simulink model "Model"  (R2020b)
settings: Solver=VariableStepAuto  StartTime=0.0  StopTime=20  MaxStep=0.1  RelTol=1e-1
values from neighbouring files (symbols this model uses):
  D = [0 ... (first row only)    [Data_clean.m]
  g = 9.81    [Data_clean.m]
  k_cart = 0.0113    [Data_clean.m]
  L = 5    [Data_clean.m]
  m = 12000    [Data_clean.m]
  M = 1000    [Data_clean.m]
  Ts = 0.1    [Data_clean.m]
undefined symbols (not defined in the file or in its folder): blk, Discrete, iA, isLTV, lastPcov, lastu, lastx, MDscale, mpc1_plant, MVscale, nCC, nu, nud, nv, nxp, ny, nym, p, RMVscale, Time, ts, uoff, X, xoff, Y, Yscale, Z
libraries: sm_lib x76, mpcsigdimcheck_private x76, nesl_utility x12, ctrlSharedLib x8, simulink_extras x5, mpclib x1
(part 5 of 8)

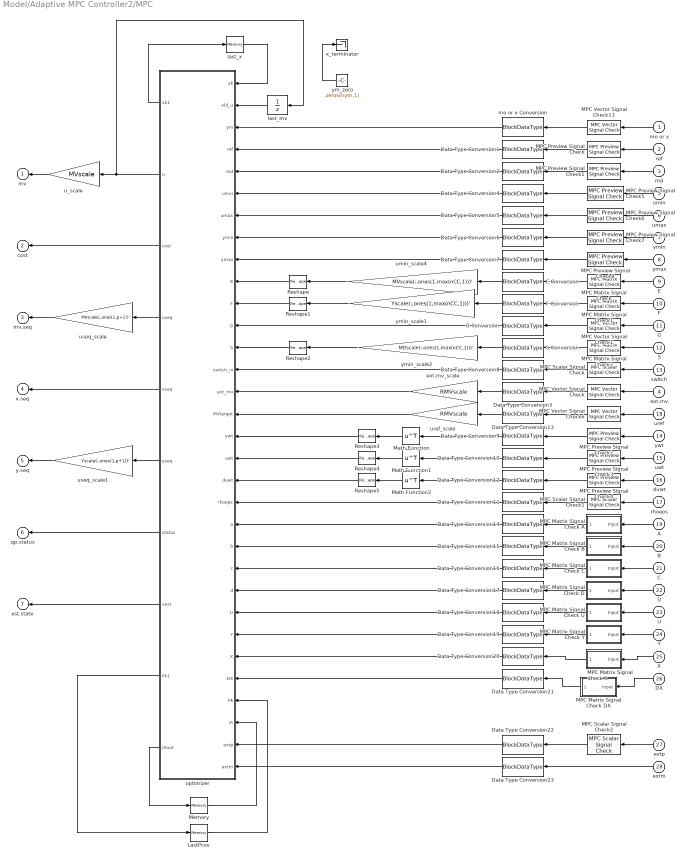
== system Model/Adaptive MPC Controller2/MPC ==
  mo or x : Inport
  ref : Inport  Port=2
  md : Inport  Port=3
  ext.mv : Inport  Port=4
  umin : Inport  Port=5
  umax : Inport  Port=6
  ymin : Inport  Port=7
  ymax : Inport  Port=8
  E : Inport  Port=9
  F : Inport  Port=10
  G : Inport  Port=11
  S : Inport  Port=12
  switch : Inport  Port=13
  ywt : Inport  Port=14
  uwt : Inport  Port=15
  duwt : Inport  Port=16
  rhoeps : Inport  Port=17
  uref : Inport  Port=18
  A : Inport  Port=19
  B : Inport  Port=20
  C : Inport  Port=21
  D : Inport  Port=22
  U : Inport  Port=23
  Y : Inport  Port=24
  X : Inport  Port=25
  DX : Inport  Port=26
  extp : Inport  Port=27
  extm : Inport  Port=28
  Data Type Conversion{1..23} (23 alike) : DataTypeConversion  OutDataTypeStr=BlockDataType
  E Conversion : DataTypeConversion  OutDataTypeStr=BlockDataType
  F Conversion : DataTypeConversion  OutDataTypeStr=BlockDataType
  G Conversion : DataTypeConversion  OutDataTypeStr=BlockDataType
  LastPcov : Memory  InitialCondition=lastPcov  InheritSampleTime=on  LinearizeAsDelay=on
  MPC Matrix Signal Check : mpcsigdimcheck_private/MPC Matrix Signal Check  blockname=blk  signalname='CustomConstraint.E'  numrow=max(nCC,1)  numcol=nu  steps=0  isLTV=0
      settings: SourceProductBaseCode=MP
  MPC Matrix Signal Check A : Subsystem  AncestorBlock=mpcsigdimcheck_private/MPC Matrix Signal Check  mask(MPCSignalDimensionCheck){blockname=blk, signalname='Model.A', numrow=nxp, numcol=nxp, steps=p, isLTV=isLTV}
      mask prompts: blockname "Block name"; signalname "Signal name"; numrow "Number of rows"; numcol "Number of columns"; steps "Number of prediction steps"; isLTV "Linear Time-Varying (LTV) plants"
      mask help: Internal use to check MPC input signal dimensions at compile time.
      mask init:
      | nrow = uint16(numrow);
      | ncol = uint16(numcol);
      | nsteps = uint16(steps);
      | isltv = uint16(isLTV);
  MPC Matrix Signal Check B : Subsystem  AncestorBlock=mpcsigdimcheck_private/MPC Matrix Signal Check  mask(MPCSignalDimensionCheck){blockname=blk, signalname='Model.B', numrow=nxp, numcol=nu+nv-1+nud, steps=p, isLTV=isLTV}
      mask prompts: blockname "Block name"; signalname "Signal name"; numrow "Number of rows"; numcol "Number of columns"; steps "Number of prediction steps"; isLTV "Linear Time-Varying (LTV) plants"
      mask help: Internal use to check MPC input signal dimensions at compile time.
      mask init:
      | nrow = uint16(numrow);
      | ncol = uint16(numcol);
      | nsteps = uint16(steps);
      | isltv = uint16(isLTV);
  MPC Matrix Signal Check C : Subsystem  AncestorBlock=mpcsigdimcheck_private/MPC Matrix Signal Check  mask(MPCSignalDimensionCheck){blockname=blk, signalname='Model.C', numrow=ny, numcol=nxp, steps=p, isLTV=isLTV}
      mask prompts: blockname "Block name"; signalname "Signal name"; numrow "Number of rows"; numcol "Number of columns"; steps "Number of prediction steps"; isLTV "Linear Time-Varying (LTV) plants"
      mask help: Internal use to check MPC input signal dimensions at compile time.
      mask init:
      | nrow = uint16(numrow);
      | ncol = uint16(numcol);
      | nsteps = uint16(steps);
      | isltv = uint16(isLTV);
  MPC Matrix Signal Check D : Subsystem  AncestorBlock=mpcsigdimcheck_private/MPC Matrix Signal Check  mask(MPCSignalDimensionCheck){blockname=blk, signalname='Model.D', numrow=ny, numcol=nu+nv-1+nud, steps=p, isLTV=isLTV}
      mask prompts: blockname "Block name"; signalname "Signal name"; numrow "Number of rows"; numcol "Number of columns"; steps "Number of prediction steps"; isLTV "Linear Time-Varying (LTV) plants"
      mask help: Internal use to check MPC input signal dimensions at compile time.
      mask init:
      | nrow = uint16(numrow);
      | ncol = uint16(numcol);
      | nsteps = uint16(steps);
      | isltv = uint16(isLTV);
  MPC Matrix Signal Check DX : Subsystem  AncestorBlock=mpcsigdimcheck_private/MPC Matrix Signal Check  mask(MPCSignalDimensionCheck){blockname=blk, signalname='Model.DX', numrow=nxp, numcol=1, steps=p, isLTV=isLTV}
      mask prompts: blockname "Block name"; signalname "Signal name"; numrow "Number of rows"; numcol "Number of columns"; steps "Number of prediction steps"; isLTV "Linear Time-Varying (LTV) plants"
      mask help: Internal use to check MPC input signal dimensions at compile time.
      mask init:
      | nrow = uint16(numrow);
      | ncol = uint16(numcol);
      | nsteps = uint16(steps);
      | isltv = uint16(isLTV);
  MPC Matrix Signal Check U : Subsystem  AncestorBlock=mpcsigdimcheck_private/MPC Matrix Signal Check  mask(MPCSignalDimensionCheck){blockname=blk, signalname='Model.U', numrow=nu+nv-1+nud, numcol=1, steps=p, isLTV=isLTV}
      mask prompts: blockname "Block name"; signalname "Signal name"; numrow "Number of rows"; numcol "Number of columns"; steps "Number of prediction steps"; isLTV "Linear Time-Varying (LTV) plants"
      mask help: Internal use to check MPC input signal dimensions at compile time.
      mask init:
      | nrow = uint16(numrow);
      | ncol = uint16(numcol);
      | nsteps = uint16(steps);
      | isltv = uint16(isLTV);
  MPC Matrix Signal Check X : Subsystem  AncestorBlock=mpcsigdimcheck_private/MPC Matrix Signal Check  mask(MPCSignalDimensionCheck){blockname=blk, signalname='Model.X', numrow=nxp, numcol=1, steps=p, isLTV=isLTV}
      mask prompts: blockname "Block name"; signalname "Signal name"; numrow "Number of rows"; numcol "Number of columns"; steps "Number of prediction steps"; isLTV "Linear Time-Varying (LTV) plants"
      mask help: Internal use to check MPC input signal dimensions at compile time.
      mask init:
      | nrow = uint16(numrow);
      | ncol = uint16(numcol);
      | nsteps = uint16(steps);
      | isltv = uint16(isLTV);
  MPC Matrix Signal Check Y : Subsystem  AncestorBlock=mpcsigdimcheck_private/MPC Matrix Signal Check  mask(MPCSignalDimensionCheck){blockname=blk, signalname='Model.Y', numrow=ny, numcol=1, steps=p, isLTV=isLTV}
      mask prompts: blockname "Block name"; signalname "Signal name"; numrow "Number of rows"; numcol "Number of columns"; steps "Number of prediction steps"; isLTV "Linear Time-Varying (LTV) plants"
      mask help: Internal use to check MPC input signal dimensions at compile time.
      mask init:
      | nrow = uint16(numrow);
      | ncol = uint16(numcol);
      | nsteps = uint16(steps);
      | isltv = uint16(isLTV);
  MPC Matrix Signal Check1 : mpcsigdimcheck_private/MPC Matrix Signal Check  blockname=blk  signalname='CustomConstraint.F'  numrow=max(nCC,1)  numcol=ny  steps=0  isLTV=0
      settings: SourceProductBaseCode=MP
  MPC Matrix Signal Check2 : mpcsigdimcheck_private/MPC Matrix Signal Check  blockname=blk  signalname='CustomConstraint.S'  numrow=max(nCC,1)  numcol=max(nv-1,1)  steps=0  isLTV=0
      settings: SourceProductBaseCode=MP
  MPC Preview Signal Check : mpcsigdimcheck_private/MPC Preview Signal Check  blockname=blk  signalname='ref'  numrow=p  numcol=ny
      settings: SourceProductBaseCode=MP
  MPC Preview Signal Check1 : mpcsigdimcheck_private/MPC Preview Signal Check  blockname=blk  signalname='md'  numrow=p+1  numcol=max(nv-1,1)
      settings: SourceProductBaseCode=MP
  MPC Preview Signal Check2 : mpcsigdimcheck_private/MPC Preview Signal Check  blockname=blk  signalname='y.wt'  numrow=p  numcol=ny
      settings: SourceProductBaseCode=MP
  MPC Preview Signal Check3 : mpcsigdimcheck_private/MPC Preview Signal Check  blockname=blk  signalname='u.wt'  numrow=p  numcol=nu
      settings: SourceProductBaseCode=MP
  MPC Preview Signal Check4 : mpcsigdimcheck_private/MPC Preview Signal Check  blockname=blk  signalname='du.wt'  numrow=p  numcol=nu
      settings: SourceProductBaseCode=MP
  MPC Preview Signal Check5 : mpcsigdimcheck_private/MPC Preview Signal Check  blockname=blk  signalname='umin'  numrow=p  numcol=nu
      settings: SourceProductBaseCode=MP
  MPC Preview Signal Check6 : mpcsigdimcheck_private/MPC Preview Signal Check  blockname=blk  signalname='umax'  numrow=p  numcol=nu
      settings: SourceProductBaseCode=MP
  MPC Preview Signal Check7 : mpcsigdimcheck_private/MPC Preview Signal Check  blockname=blk  signalname='ymin'  numrow=p  numcol=ny
      settings: SourceProductBaseCode=MP
  MPC Preview Signal Check8 : mpcsigdimcheck_private/MPC Preview Signal Check  blockname=blk  signalname='ymax'  numrow=p  numcol=ny
      settings: SourceProductBaseCode=MP
  MPC Scalar Signal Check : mpcsigdimcheck_private/MPC Scalar Signal Check  blockname=blk  signalname='switch'
      settings: SourceProductBaseCode=MP
  MPC Scalar Signal Check1 : mpcsigdimcheck_private/MPC Scalar Signal Check  blockname=blk  signalname='ecr.wt'
      settings: SourceProductBaseCode=MP
  MPC Scalar Signal Check2 : mpcsigdimcheck_private/MPC Scalar Signal Check  blockname=blk  signalname='p'
      settings: SourceProductBaseCode=MP
  MPC Vector Signal Check : mpcsigdimcheck_private/MPC Vector Signal Check  blockname=blk  signalname='ext.mv'  num=nu  vectortype=Any
      settings: SourceProductBaseCode=MP
  MPC Vector Signal Check1 : mpcsigdimcheck_private/MPC Vector Signal Check  blockname=blk  signalname='CustomConstraint.G'  num=max(nCC,1)  vectortype=Column
      settings: SourceProductBaseCode=MP
  MPC Vector Signal Check11 : mpcsigdimcheck_private/MPC Vector Signal Check  blockname=blk  signalname=strmoorx  num=nmoorx  vectortype=Any
      settings: SourceProductBaseCode=MP
  MPC Vector Signal Check6 : mpcsigdimcheck_private/MPC Vector Signal Check  blockname=blk  signalname='mv.target'  num=nu  vectortype=Any
      settings: SourceProductBaseCode=MP
  Math Function : Math  Operator=transpose  SignedPower=on  SaturateOnIntegerOverflow=on
  Math Function1 : Math  Operator=transpose  SignedPower=on  SaturateOnIntegerOverflow=on
  Math Function2 : Math  Operator=transpose  SignedPower=on  SaturateOnIntegerOverflow=on
  Memory : Memory  InitialCondition=iA  InheritSampleTime=on  LinearizeAsDelay=on
  Reshape : Reshape  OutputDimensionality=Customize  OutputDimensions=double([max(nCC,1),nu])
  Reshape1 : Reshape  OutputDimensionality=Customize  OutputDimensions=double([max(nCC,1),ny])
  Reshape2 : Reshape  OutputDimensionality=Customize  OutputDimensions=double([max(nCC,1),max(nv-1,1)])
  Reshape3 : Reshape  OutputDimensionality=Column vector (2-D)
  Reshape4 : Reshape  OutputDimensionality=Column vector (2-D)
  Reshape5 : Reshape  OutputDimensionality=Column vector (2-D)
  S Conversion : DataTypeConversion  OutDataTypeStr=BlockDataType
  ext.mv_scale : Gain  Gain=RMVscale  SampleTime=ts
  last_mv : UnitDelay  InitialCondition=lastu+uoff  SampleTime=ts  HasFrameUpgradeWarning=on
  last_x : Memory  InitialCondition=lastx+xoff  InheritSampleTime=on  LinearizeAsDelay=on
  mo or x Conversion : DataTypeConversion  OutDataTypeStr=BlockDataType
  optimizer : Subsystem  Variant=on  VariantControlMode=label  VariantControl=Variant1  LabelModeActiveChoice=FixedHorizon
  u_scale : Gain  Gain=MVscale  SampleTime=ts
  umin_scale4 : Gain  Gain=MVscale(:,ones(1,max(nCC,1)))'  SampleTime=ts
  uref_scale : Gain  Gain=RMVscale  SampleTime=ts
  useq_scale : Gain  Gain=MVscale(:,ones(1,p+1))'  SampleTime=ts
  useq_scale1 : Gain  Gain=Yscale(:,ones(1,p+1))'  SampleTime=ts
  x_terminator : Terminator
  ym_zero : Constant  Value=zeros(nym,1)  OutDataTypeStr=BlockDataType
  ymin_scale1 : Gain  Gain=Yscale(:,ones(1,max(nCC,1)))'  SampleTime=ts
  ymin_scale2 : Gain  Gain=MDscale(:,ones(1,max(nCC,1)))'  SampleTime=ts
  mv : Outport  OutDataTypeStr=BlockDataType  VectorParamsAs1DForOutWhenUnconnected=off
  cost : Outport  Port=2  OutDataTypeStr=BlockDataType  VectorParamsAs1DForOutWhenUnconnected=off
  mv.seq : Outport  Port=3  OutDataTypeStr=BlockDataType  VectorParamsAs1DForOutWhenUnconnected=off
  x.seq : Outport  Port=4  OutDataTypeStr=BlockDataType  VectorParamsAs1DForOutWhenUnconnected=off
  y.seq : Outport  Port=5  OutDataTypeStr=BlockDataType  VectorParamsAs1DForOutWhenUnconnected=off
  qp.status : Outport  Port=6  OutDataTypeStr=BlockDataType  VectorParamsAs1DForOutWhenUnconnected=off
  est.state : Outport  Port=7  OutDataTypeStr=BlockDataType  VectorParamsAs1DForOutWhenUnconnected=off
  wires:
  MPC Scalar Signal Check2/1 -> Data Type Conversion22/1
  extm/1 -> Data Type Conversion23/1
  extp/1 -> MPC Scalar Signal Check2/1
  Data Type Conversion23/1 -> optimizer/32(extm)
  Data Type Conversion22/1 -> optimizer/31(extp)
  optimizer/10(" iAout") -> Memory/1
  optimizer/9(" Pk1") -> LastPcov/1
  optimizer/8(" xest") -> est.state/1
  optimizer/7(" status") -> qp.status/1
  optimizer/6(" yseq") -> useq_scale1/1
  optimizer/5(" xseq") -> x.seq/1
  optimizer/4(" useq") -> useq_scale/1
  optimizer/3(" cost") -> cost/1
  optimizer/2(" u") -> last_mv/1, u_scale/1
  optimizer/1(" xk1") -> last_x/1
  Memory/1 -> optimizer/30("iA ")
  LastPcov/1 -> optimizer/29("Pk ")
  Data Type Conversion21/1 -> optimizer/28("DX ")
  Data Type Conversion20/1 -> optimizer/27("X ")
  Data Type Conversion19/1 -> optimizer/26("Y ")
  Data Type Conversion18/1 -> optimizer/25("U ")
  Data Type Conversion17/1 -> optimizer/24("d ")
  Data Type Conversion16/1 -> optimizer/23("c ")
  Data Type Conversion15/1 -> optimizer/22("b ")
  Data Type Conversion14/1 -> optimizer/21("a ")
  Data Type Conversion11/1 -> optimizer/20("rhoeps ")
  Reshape5/1 -> optimizer/19("duwt ")
  Reshape4/1 -> optimizer/18("uwt ")
  Reshape3/1 -> optimizer/17("ywt ")
  uref_scale/1 -> optimizer/16("MVtarget ")
  ext.mv_scale/1 -> optimizer/15("ext_mv ")
  Data Type Conversion8/1 -> optimizer/14("switch_in ")
  Reshape2/1 -> optimizer/13("S ")
  G Conversion/1 -> optimizer/12("G ")
  Reshape1/1 -> optimizer/11("F ")
  Reshape/1 -> optimizer/10("E ")
  Data Type Conversion7/1 -> optimizer/9("ymax ")
  Data Type Conversion6/1 -> optimizer/8("ymin ")
  Data Type Conversion5/1 -> optimizer/7("umax ")
  Data Type Conversion4/1 -> optimizer/6("umin ")
  Data Type Conversion2/1 -> optimizer/5("md ")
  Data Type Conversion1/1 -> optimizer/4("ref ")
  mo or x Conversion/1 -> optimizer/3("ym ")
  last_mv/1 -> optimizer/2("old_u ")
  last_x/1 -> optimizer/1("xk ")
  useq_scale1/1 -> y.seq/1
  Math Function2/1 -> Reshape5/1
  Math Function1/1 -> Reshape4/1
  Math Function/1 -> Reshape3/1
  MPC Matrix Signal Check1/1 -> F Conversion/1
  umin_scale4/1 -> Reshape/1
  ymin_scale1/1 -> Reshape1/1
  G/1 -> MPC Vector Signal Check1/1
  F/1 -> MPC Matrix Signal Check1/1
  E Conversion/1 -> umin_scale4/1
  ymin_scale2/1 -> Reshape2/1
  MPC Matrix Signal Check/1 -> E Conversion/1
  S/1 -> MPC Matrix Signal Check2/1
  E/1 -> MPC Matrix Signal Check/1
  MPC Matrix Signal Check2/1 -> S Conversion/1
  MPC Vector Signal Check1/1 -> G Conversion/1
  S Conversion/1 -> ymin_scale2/1
  F Conversion/1 -> ymin_scale1/1
  MPC Matrix Signal Check DX/1(Output) -> Data Type Conversion21/1
  MPC Matrix Signal Check X/1(Output) -> Data Type Conversion20/1
  MPC Matrix Signal Check Y/1(Output) -> Data Type Conversion19/1
  MPC Matrix Signal Check U/1(Output) -> Data Type Conversion18/1
  MPC Matrix Signal Check D/1(Output) -> Data Type Conversion17/1
  MPC Matrix Signal Check C/1(Output) -> Data Type Conversion16/1
  MPC Matrix Signal Check B/1(Output) -> Data Type Conversion15/1
  MPC Matrix Signal Check A/1(Output) -> Data Type Conversion14/1
  MPC Scalar Signal Check1/1 -> Data Type Conversion11/1
  MPC Preview Signal Check4/1 -> Data Type Conversion12/1
  MPC Preview Signal Check3/1 -> Data Type Conversion10/1
  MPC Preview Signal Check2/1 -> Data Type Conversion9/1
  MPC Vector Signal Check6/1 -> Data Type Conversion13/1
  MPC Vector Signal Check/1 -> Data Type Conversion3/1
  MPC Scalar Signal Check/1 -> Data Type Conversion8/1
  MPC Preview Signal Check8/1 -> Data Type Conversion7/1
  MPC Preview Signal Check7/1 -> Data Type Conversion6/1
  MPC Preview Signal Check6/1 -> Data Type Conversion5/1
  MPC Preview Signal Check5/1 -> Data Type Conversion4/1
  MPC Preview Signal Check1/1 -> Data Type Conversion2/1
  MPC Preview Signal Check/1 -> Data Type Conversion1/1
  MPC Vector Signal Check11/1 -> mo or x Conversion/1
  useq_scale/1 -> mv.seq/1
  u_scale/1 -> mv/1
  DX/1 -> MPC Matrix Signal Check DX/1(Input)
  X/1 -> MPC Matrix Signal Check X/1(Input)
  Y/1 -> MPC Matrix Signal Check Y/1(Input)
  U/1 -> MPC Matrix Signal Check U/1(Input)
  D/1 -> MPC Matrix Signal Check D/1(Input)
  C/1 -> MPC Matrix Signal Check C/1(Input)
  B/1 -> MPC Matrix Signal Check B/1(Input)
  A/1 -> MPC Matrix Signal Check A/1(Input)
  md/1 -> MPC Preview Signal Check1/1
  umin/1 -> MPC Preview Signal Check5/1
  umax/1 -> MPC Preview Signal Check6/1
  ymin/1 -> MPC Preview Signal Check7/1
  ymax/1 -> MPC Preview Signal Check8/1
  switch/1 -> MPC Scalar Signal Check/1
  ext.mv/1 -> MPC Vector Signal Check/1
  Data Type Conversion3/1 -> ext.mv_scale/1
  ref/1 -> MPC Preview Signal Check/1
  mo or x/1 -> MPC Vector Signal Check11/1
  ywt/1 -> MPC Preview Signal Check2/1
  uwt/1 -> MPC Preview Signal Check3/1
  Data Type Conversion9/1 -> Math Function/1
  Data Type Conversion12/1 -> Math Function2/1
  rhoeps/1 -> MPC Scalar Signal Check1/1
  duwt/1 -> MPC Preview Signal Check4/1
  Data Type Conversion10/1 -> Math Function1/1
  uref/1 -> MPC Vector Signal Check6/1
  Data Type Conversion13/1 -> uref_scale/1
  ym_zero/1 -> x_terminator/1

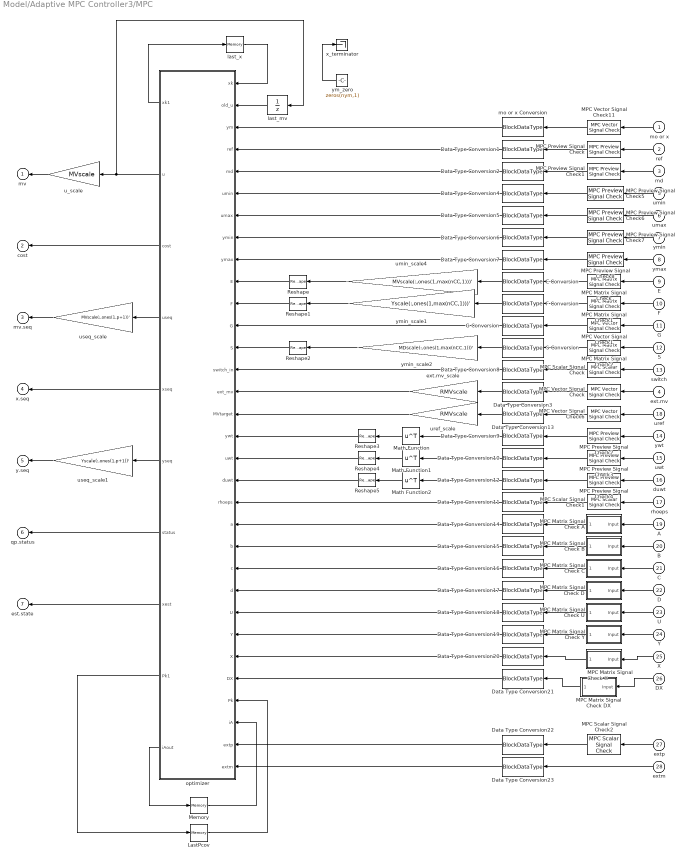
== system Model/Adaptive MPC Controller3/MPC ==
  mo or x : Inport
  ref : Inport  Port=2
  md : Inport  Port=3
  ext.mv : Inport  Port=4
  umin : Inport  Port=5
  umax : Inport  Port=6
  ymin : Inport  Port=7
  ymax : Inport  Port=8
  E : Inport  Port=9
  F : Inport  Port=10
  G : Inport  Port=11
  S : Inport  Port=12
  switch : Inport  Port=13
  ywt : Inport  Port=14
  uwt : Inport  Port=15
  duwt : Inport  Port=16
  rhoeps : Inport  Port=17
  uref : Inport  Port=18
  A : Inport  Port=19
  B : Inport  Port=20
  C : Inport  Port=21
  D : Inport  Port=22
  U : Inport  Port=23
  Y : Inport  Port=24
  X : Inport  Port=25
  DX : Inport  Port=26
  extp : Inport  Port=27
  extm : Inport  Port=28
  Data Type Conversion{1..23} (23 alike) : DataTypeConversion  OutDataTypeStr=BlockDataType
  E Conversion : DataTypeConversion  OutDataTypeStr=BlockDataType
  F Conversion : DataTypeConversion  OutDataTypeStr=BlockDataType
  G Conversion : DataTypeConversion  OutDataTypeStr=BlockDataType
  LastPcov : Memory  InitialCondition=lastPcov  InheritSampleTime=on  LinearizeAsDelay=on
  MPC Matrix Signal Check : mpcsigdimcheck_private/MPC Matrix Signal Check  blockname=blk  signalname='CustomConstraint.E'  numrow=max(nCC,1)  numcol=nu  steps=0  isLTV=0
      settings: SourceProductBaseCode=MP
  MPC Matrix Signal Check A : Subsystem  AncestorBlock=mpcsigdimcheck_private/MPC Matrix Signal Check  mask(MPCSignalDimensionCheck){blockname=blk, signalname='Model.A', numrow=nxp, numcol=nxp, steps=p, isLTV=isLTV}
      mask prompts: blockname "Block name"; signalname "Signal name"; numrow "Number of rows"; numcol "Number of columns"; steps "Number of prediction steps"; isLTV "Linear Time-Varying (LTV) plants"
      mask help: Internal use to check MPC input signal dimensions at compile time.
      mask init:
      | nrow = uint16(numrow);
      | ncol = uint16(numcol);
      | nsteps = uint16(steps);
      | isltv = uint16(isLTV);
  MPC Matrix Signal Check B : Subsystem  AncestorBlock=mpcsigdimcheck_private/MPC Matrix Signal Check  mask(MPCSignalDimensionCheck){blockname=blk, signalname='Model.B', numrow=nxp, numcol=nu+nv-1+nud, steps=p, isLTV=isLTV}
      mask prompts: blockname "Block name"; signalname "Signal name"; numrow "Number of rows"; numcol "Number of columns"; steps "Number of prediction steps"; isLTV "Linear Time-Varying (LTV) plants"
      mask help: Internal use to check MPC input signal dimensions at compile time.
      mask init:
      | nrow = uint16(numrow);
      | ncol = uint16(numcol);
      | nsteps = uint16(steps);
      | isltv = uint16(isLTV);
  MPC Matrix Signal Check C : Subsystem  AncestorBlock=mpcsigdimcheck_private/MPC Matrix Signal Check  mask(MPCSignalDimensionCheck){blockname=blk, signalname='Model.C', numrow=ny, numcol=nxp, steps=p, isLTV=isLTV}
      mask prompts: blockname "Block name"; signalname "Signal name"; numrow "Number of rows"; numcol "Number of columns"; steps "Number of prediction steps"; isLTV "Linear Time-Varying (LTV) plants"
      mask help: Internal use to check MPC input signal dimensions at compile time.
      mask init:
      | nrow = uint16(numrow);
      | ncol = uint16(numcol);
      | nsteps = uint16(steps);
      | isltv = uint16(isLTV);
  MPC Matrix Signal Check D : Subsystem  AncestorBlock=mpcsigdimcheck_private/MPC Matrix Signal Check  mask(MPCSignalDimensionCheck){blockname=blk, signalname='Model.D', numrow=ny, numcol=nu+nv-1+nud, steps=p, isLTV=isLTV}
      mask prompts: blockname "Block name"; signalname "Signal name"; numrow "Number of rows"; numcol "Number of columns"; steps "Number of prediction steps"; isLTV "Linear Time-Varying (LTV) plants"
      mask help: Internal use to check MPC input signal dimensions at compile time.
      mask init:
      | nrow = uint16(numrow);
      | ncol = uint16(numcol);
      | nsteps = uint16(steps);
      | isltv = uint16(isLTV);
  MPC Matrix Signal Check DX : Subsystem  AncestorBlock=mpcsigdimcheck_private/MPC Matrix Signal Check  mask(MPCSignalDimensionCheck){blockname=blk, signalname='Model.DX', numrow=nxp, numcol=1, steps=p, isLTV=isLTV}
      mask prompts: blockname "Block name"; signalname "Signal name"; numrow "Number of rows"; numcol "Number of columns"; steps "Number of prediction steps"; isLTV "Linear Time-Varying (LTV) plants"
      mask help: Internal use to check MPC input signal dimensions at compile time.
      mask init:
      | nrow = uint16(numrow);
      | ncol = uint16(numcol);
      | nsteps = uint16(steps);
      | isltv = uint16(isLTV);
  MPC Matrix Signal Check U : Subsystem  AncestorBlock=mpcsigdimcheck_private/MPC Matrix Signal Check  mask(MPCSignalDimensionCheck){blockname=blk, signalname='Model.U', numrow=nu+nv-1+nud, numcol=1, steps=p, isLTV=isLTV}
      mask prompts: blockname "Block name"; signalname "Signal name"; numrow "Number of rows"; numcol "Number of columns"; steps "Number of prediction steps"; isLTV "Linear Time-Varying (LTV) plants"
      mask help: Internal use to check MPC input signal dimensions at compile time.
      mask init:
      | nrow = uint16(numrow);
      | ncol = uint16(numcol);
      | nsteps = uint16(steps);
      | isltv = uint16(isLTV);
  MPC Matrix Signal Check X : Subsystem  AncestorBlock=mpcsigdimcheck_private/MPC Matrix Signal Check  mask(MPCSignalDimensionCheck){blockname=blk, signalname='Model.X', numrow=nxp, numcol=1, steps=p, isLTV=isLTV}
      mask prompts: blockname "Block name"; signalname "Signal name"; numrow "Number of rows"; numcol "Number of columns"; steps "Number of prediction steps"; isLTV "Linear Time-Varying (LTV) plants"
      mask help: Internal use to check MPC input signal dimensions at compile time.
      mask init:
      | nrow = uint16(numrow);
      | ncol = uint16(numcol);
      | nsteps = uint16(steps);
      | isltv = uint16(isLTV);
  MPC Matrix Signal Check Y : Subsystem  AncestorBlock=mpcsigdimcheck_private/MPC Matrix Signal Check  mask(MPCSignalDimensionCheck){blockname=blk, signalname='Model.Y', numrow=ny, numcol=1, steps=p, isLTV=isLTV}
      mask prompts: blockname "Block name"; signalname "Signal name"; numrow "Number of rows"; numcol "Number of columns"; steps "Number of prediction steps"; isLTV "Linear Time-Varying (LTV) plants"
      mask help: Internal use to check MPC input signal dimensions at compile time.
      mask init:
      | nrow = uint16(numrow);
      | ncol = uint16(numcol);
      | nsteps = uint16(steps);
      | isltv = uint16(isLTV);
  MPC Matrix Signal Check1 : mpcsigdimcheck_private/MPC Matrix Signal Check  blockname=blk  signalname='CustomConstraint.F'  numrow=max(nCC,1)  numcol=ny  steps=0  isLTV=0
      settings: SourceProductBaseCode=MP
  MPC Matrix Signal Check2 : mpcsigdimcheck_private/MPC Matrix Signal Check  blockname=blk  signalname='CustomConstraint.S'  numrow=max(nCC,1)  numcol=max(nv-1,1)  steps=0  isLTV=0
      settings: SourceProductBaseCode=MP
  MPC Preview Signal Check : mpcsigdimcheck_private/MPC Preview Signal Check  blockname=blk  signalname='ref'  numrow=p  numcol=ny
      settings: SourceProductBaseCode=MP
  MPC Preview Signal Check1 : mpcsigdimcheck_private/MPC Preview Signal Check  blockname=blk  signalname='md'  numrow=p+1  numcol=max(nv-1,1)
      settings: SourceProductBaseCode=MP
  MPC Preview Signal Check2 : mpcsigdimcheck_private/MPC Preview Signal Check  blockname=blk  signalname='y.wt'  numrow=p  numcol=ny
      settings: SourceProductBaseCode=MP
  MPC Preview Signal Check3 : mpcsigdimcheck_private/MPC Preview Signal Check  blockname=blk  signalname='u.wt'  numrow=p  numcol=nu
      settings: SourceProductBaseCode=MP
  MPC Preview Signal Check4 : mpcsigdimcheck_private/MPC Preview Signal Check  blockname=blk  signalname='du.wt'  numrow=p  numcol=nu
      settings: SourceProductBaseCode=MP
  MPC Preview Signal Check5 : mpcsigdimcheck_private/MPC Preview Signal Check  blockname=blk  signalname='umin'  numrow=p  numcol=nu
      settings: SourceProductBaseCode=MP
  MPC Preview Signal Check6 : mpcsigdimcheck_private/MPC Preview Signal Check  blockname=blk  signalname='umax'  numrow=p  numcol=nu
      settings: SourceProductBaseCode=MP
  MPC Preview Signal Check7 : mpcsigdimcheck_private/MPC Preview Signal Check  blockname=blk  signalname='ymin'  numrow=p  numcol=ny
      settings: SourceProductBaseCode=MP
  MPC Preview Signal Check8 : mpcsigdimcheck_private/MPC Preview Signal Check  blockname=blk  signalname='ymax'  numrow=p  numcol=ny
      settings: SourceProductBaseCode=MP
  MPC Scalar Signal Check : mpcsigdimcheck_private/MPC Scalar Signal Check  blockname=blk  signalname='switch'
      settings: SourceProductBaseCode=MP
  MPC Scalar Signal Check1 : mpcsigdimcheck_private/MPC Scalar Signal Check  blockname=blk  signalname='ecr.wt'
      settings: SourceProductBaseCode=MP
  MPC Scalar Signal Check2 : mpcsigdimcheck_private/MPC Scalar Signal Check  blockname=blk  signalname='p'
      settings: SourceProductBaseCode=MP
  MPC Vector Signal Check : mpcsigdimcheck_private/MPC Vector Signal Check  blockname=blk  signalname='ext.mv'  num=nu  vectortype=Any
      settings: SourceProductBaseCode=MP
  MPC Vector Signal Check1 : mpcsigdimcheck_private/MPC Vector Signal Check  blockname=blk  signalname='CustomConstraint.G'  num=max(nCC,1)  vectortype=Column
      settings: SourceProductBaseCode=MP
  MPC Vector Signal Check11 : mpcsigdimcheck_private/MPC Vector Signal Check  blockname=blk  signalname=strmoorx  num=nmoorx  vectortype=Any
      settings: SourceProductBaseCode=MP
  MPC Vector Signal Check6 : mpcsigdimcheck_private/MPC Vector Signal Check  blockname=blk  signalname='mv.target'  num=nu  vectortype=Any
      settings: SourceProductBaseCode=MP
  Math Function : Math  Operator=transpose  SignedPower=on  SaturateOnIntegerOverflow=on
  Math Function1 : Math  Operator=transpose  SignedPower=on  SaturateOnIntegerOverflow=on
  Math Function2 : Math  Operator=transpose  SignedPower=on  SaturateOnIntegerOverflow=on
  Memory : Memory  InitialCondition=iA  InheritSampleTime=on  LinearizeAsDelay=on
  Reshape : Reshape  OutputDimensionality=Customize  OutputDimensions=double([max(nCC,1),nu])
  Reshape1 : Reshape  OutputDimensionality=Customize  OutputDimensions=double([max(nCC,1),ny])
  Reshape2 : Reshape  OutputDimensionality=Customize  OutputDimensions=double([max(nCC,1),max(nv-1,1)])
  Reshape3 : Reshape  OutputDimensionality=Column vector (2-D)
  Reshape4 : Reshape  OutputDimensionality=Column vector (2-D)
  Reshape5 : Reshape  OutputDimensionality=Column vector (2-D)
  S Conversion : DataTypeConversion  OutDataTypeStr=BlockDataType
  ext.mv_scale : Gain  Gain=RMVscale  SampleTime=ts
  last_mv : UnitDelay  InitialCondition=lastu+uoff  SampleTime=ts  HasFrameUpgradeWarning=on
  last_x : Memory  InitialCondition=lastx+xoff  InheritSampleTime=on  LinearizeAsDelay=on
  mo or x Conversion : DataTypeConversion  OutDataTypeStr=BlockDataType
  optimizer : Subsystem  Variant=on  VariantControlMode=label  VariantControl=Variant1  LabelModeActiveChoice=FixedHorizon
  u_scale : Gain  Gain=MVscale  SampleTime=ts
  umin_scale4 : Gain  Gain=MVscale(:,ones(1,max(nCC,1)))'  SampleTime=ts
  uref_scale : Gain  Gain=RMVscale  SampleTime=ts
  useq_scale : Gain  Gain=MVscale(:,ones(1,p+1))'  SampleTime=ts
  useq_scale1 : Gain  Gain=Yscale(:,ones(1,p+1))'  SampleTime=ts
  x_terminator : Terminator
  ym_zero : Constant  Value=zeros(nym,1)  OutDataTypeStr=BlockDataType
  ymin_scale1 : Gain  Gain=Yscale(:,ones(1,max(nCC,1)))'  SampleTime=ts
  ymin_scale2 : Gain  Gain=MDscale(:,ones(1,max(nCC,1)))'  SampleTime=ts
  mv : Outport  OutDataTypeStr=BlockDataType  VectorParamsAs1DForOutWhenUnconnected=off
  cost : Outport  Port=2  OutDataTypeStr=BlockDataType  VectorParamsAs1DForOutWhenUnconnected=off
  mv.seq : Outport  Port=3  OutDataTypeStr=BlockDataType  VectorParamsAs1DForOutWhenUnconnected=off
  x.seq : Outport  Port=4  OutDataTypeStr=BlockDataType  VectorParamsAs1DForOutWhenUnconnected=off
  y.seq : Outport  Port=5  OutDataTypeStr=BlockDataType  VectorParamsAs1DForOutWhenUnconnected=off
  qp.status : Outport  Port=6  OutDataTypeStr=BlockDataType  VectorParamsAs1DForOutWhenUnconnected=off
  est.state : Outport  Port=7  OutDataTypeStr=BlockDataType  VectorParamsAs1DForOutWhenUnconnected=off
  wires:
  MPC Scalar Signal Check2/1 -> Data Type Conversion22/1
  extm/1 -> Data Type Conversion23/1
  extp/1 -> MPC Scalar Signal Check2/1
  Data Type Conversion23/1 -> optimizer/32(extm)
  Data Type Conversion22/1 -> optimizer/31(extp)
  optimizer/10(" iAout") -> Memory/1
  optimizer/9(" Pk1") -> LastPcov/1
  optimizer/8(" xest") -> est.state/1
  optimizer/7(" status") -> qp.status/1
  optimizer/6(" yseq") -> useq_scale1/1
  optimizer/5(" xseq") -> x.seq/1
  optimizer/4(" useq") -> useq_scale/1
  optimizer/3(" cost") -> cost/1
  optimizer/2(" u") -> last_mv/1, u_scale/1
  optimizer/1(" xk1") -> last_x/1
  Memory/1 -> optimizer/30("iA ")
  LastPcov/1 -> optimizer/29("Pk ")
  Data Type Conversion21/1 -> optimizer/28("DX ")
  Data Type Conversion20/1 -> optimizer/27("X ")
  Data Type Conversion19/1 -> optimizer/26("Y ")
  Data Type Conversion18/1 -> optimizer/25("U ")
  Data Type Conversion17/1 -> optimizer/24("d ")
  Data Type Conversion16/1 -> optimizer/23("c ")
  Data Type Conversion15/1 -> optimizer/22("b ")
  Data Type Conversion14/1 -> optimizer/21("a ")
  Data Type Conversion11/1 -> optimizer/20("rhoeps ")
  Reshape5/1 -> optimizer/19("duwt ")
  Reshape4/1 -> optimizer/18("uwt ")
  Reshape3/1 -> optimizer/17("ywt ")
  uref_scale/1 -> optimizer/16("MVtarget ")
  ext.mv_scale/1 -> optimizer/15("ext_mv ")
  Data Type Conversion8/1 -> optimizer/14("switch_in ")
  Reshape2/1 -> optimizer/13("S ")
  G Conversion/1 -> optimizer/12("G ")
  Reshape1/1 -> optimizer/11("F ")
  Reshape/1 -> optimizer/10("E ")
  Data Type Conversion7/1 -> optimizer/9("ymax ")
  Data Type Conversion6/1 -> optimizer/8("ymin ")
  Data Type Conversion5/1 -> optimizer/7("umax ")
  Data Type Conversion4/1 -> optimizer/6("umin ")
  Data Type Conversion2/1 -> optimizer/5("md ")
  Data Type Conversion1/1 -> optimizer/4("ref ")
  mo or x Conversion/1 -> optimizer/3("ym ")
  last_mv/1 -> optimizer/2("old_u ")
  last_x/1 -> optimizer/1("xk ")
  useq_scale1/1 -> y.seq/1
  Math Function2/1 -> Reshape5/1
  Math Function1/1 -> Reshape4/1
  Math Function/1 -> Reshape3/1
  MPC Matrix Signal Check1/1 -> F Conversion/1
  umin_scale4/1 -> Reshape/1
  ymin_scale1/1 -> Reshape1/1
  G/1 -> MPC Vector Signal Check1/1
  F/1 -> MPC Matrix Signal Check1/1
  E Conversion/1 -> umin_scale4/1
  ymin_scale2/1 -> Reshape2/1
  MPC Matrix Signal Check/1 -> E Conversion/1
  S/1 -> MPC Matrix Signal Check2/1
  E/1 -> MPC Matrix Signal Check/1
  MPC Matrix Signal Check2/1 -> S Conversion/1
  MPC Vector Signal Check1/1 -> G Conversion/1
  S Conversion/1 -> ymin_scale2/1
  F Conversion/1 -> ymin_scale1/1
  MPC Matrix Signal Check DX/1(Output) -> Data Type Conversion21/1
  MPC Matrix Signal Check X/1(Output) -> Data Type Conversion20/1
  MPC Matrix Signal Check Y/1(Output) -> Data Type Conversion19/1
  MPC Matrix Signal Check U/1(Output) -> Data Type Conversion18/1
  MPC Matrix Signal Check D/1(Output) -> Data Type Conversion17/1
  MPC Matrix Signal Check C/1(Output) -> Data Type Conversion16/1
  MPC Matrix Signal Check B/1(Output) -> Data Type Conversion15/1
  MPC Matrix Signal Check A/1(Output) -> Data Type Conversion14/1
  MPC Scalar Signal Check1/1 -> Data Type Conversion11/1
  MPC Preview Signal Check4/1 -> Data Type Conversion12/1
  MPC Preview Signal Check3/1 -> Data Type Conversion10/1
  MPC Preview Signal Check2/1 -> Data Type Conversion9/1
  MPC Vector Signal Check6/1 -> Data Type Conversion13/1
  MPC Vector Signal Check/1 -> Data Type Conversion3/1
  MPC Scalar Signal Check/1 -> Data Type Conversion8/1
  MPC Preview Signal Check8/1 -> Data Type Conversion7/1
  MPC Preview Signal Check7/1 -> Data Type Conversion6/1
  MPC Preview Signal Check6/1 -> Data Type Conversion5/1
  MPC Preview Signal Check5/1 -> Data Type Conversion4/1
  MPC Preview Signal Check1/1 -> Data Type Conversion2/1
  MPC Preview Signal Check/1 -> Data Type Conversion1/1
  MPC Vector Signal Check11/1 -> mo or x Conversion/1
  useq_scale/1 -> mv.seq/1
  u_scale/1 -> mv/1
  DX/1 -> MPC Matrix Signal Check DX/1(Input)
  X/1 -> MPC Matrix Signal Check X/1(Input)
  Y/1 -> MPC Matrix Signal Check Y/1(Input)
  U/1 -> MPC Matrix Signal Check U/1(Input)
  D/1 -> MPC Matrix Signal Check D/1(Input)
  C/1 -> MPC Matrix Signal Check C/1(Input)
  B/1 -> MPC Matrix Signal Check B/1(Input)
  A/1 -> MPC Matrix Signal Check A/1(Input)
  md/1 -> MPC Preview Signal Check1/1
  umin/1 -> MPC Preview Signal Check5/1
  umax/1 -> MPC Preview Signal Check6/1
  ymin/1 -> MPC Preview Signal Check7/1
  ymax/1 -> MPC Preview Signal Check8/1
  switch/1 -> MPC Scalar Signal Check/1
  ext.mv/1 -> MPC Vector Signal Check/1
  Data Type Conversion3/1 -> ext.mv_scale/1
  ref/1 -> MPC Preview Signal Check/1
  mo or x/1 -> MPC Vector Signal Check11/1
  ywt/1 -> MPC Preview Signal Check2/1
  uwt/1 -> MPC Preview Signal Check3/1
  Data Type Conversion9/1 -> Math Function/1
  Data Type Conversion12/1 -> Math Function2/1
  rhoeps/1 -> MPC Scalar Signal Check1/1
  duwt/1 -> MPC Preview Signal Check4/1
  Data Type Conversion10/1 -> Math Function1/1
  uref/1 -> MPC Vector Signal Check6/1
  Data Type Conversion13/1 -> uref_scale/1
  ym_zero/1 -> x_terminator/1

== system Model/Adaptive MPC Controller/MPC/MPC Matrix Signal Check A ==
  Input : Inport
  Matrix Dimension Check : S-Function  FunctionName=mpcMatrixSignalCheck  Parameters=blockname, signalname, nrow, ncol, nsteps, isltv  SFunctionDeploymentMode=off  EnableBusSupport=off
  Signal Specification : SignalSpecification  Dimensions=[4 4]
  Output : Outport  VectorParamsAs1DForOutWhenUnconnected=off
  wires:
  Input/1 -> Output/1, Signal Specification/1
  Signal Specification/1 -> Matrix Dimension Check/1

== system Model/Adaptive MPC Controller/MPC/MPC Matrix Signal Check B ==
  Input : Inport
  Matrix Dimension Check : S-Function  FunctionName=mpcMatrixSignalCheck  Parameters=blockname, signalname, nrow, ncol, nsteps, isltv  SFunctionDeploymentMode=off  EnableBusSupport=off
  Signal Specification : SignalSpecification  Dimensions=[4 1]
  Output : Outport  VectorParamsAs1DForOutWhenUnconnected=off
  wires:
  Input/1 -> Output/1, Signal Specification/1
  Signal Specification/1 -> Matrix Dimension Check/1

== system Model/Adaptive MPC Controller/MPC/MPC Matrix Signal Check C ==
  Input : Inport
  Matrix Dimension Check : S-Function  FunctionName=mpcMatrixSignalCheck  Parameters=blockname, signalname, nrow, ncol, nsteps, isltv  SFunctionDeploymentMode=off  EnableBusSupport=off
  Signal Specification : SignalSpecification  Dimensions=[4 4]
  Output : Outport  VectorParamsAs1DForOutWhenUnconnected=off
  wires:
  Input/1 -> Output/1, Signal Specification/1
  Signal Specification/1 -> Matrix Dimension Check/1

== system Model/Adaptive MPC Controller/MPC/MPC Matrix Signal Check D ==
  Input : Inport
  Matrix Dimension Check : S-Function  FunctionName=mpcMatrixSignalCheck  Parameters=blockname, signalname, nrow, ncol, nsteps, isltv  SFunctionDeploymentMode=off  EnableBusSupport=off
  Signal Specification : SignalSpecification  Dimensions=[4 1]
  Output : Outport  VectorParamsAs1DForOutWhenUnconnected=off
  wires:
  Input/1 -> Output/1, Signal Specification/1
  Signal Specification/1 -> Matrix Dimension Check/1

== system Model/Adaptive MPC Controller/MPC/MPC Matrix Signal Check DX ==
  Input : Inport
  Matrix Dimension Check : S-Function  FunctionName=mpcMatrixSignalCheck  Parameters=blockname, signalname, nrow, ncol, nsteps, isltv  SFunctionDeploymentMode=off  EnableBusSupport=off
  Signal Specification : SignalSpecification  Dimensions=[4 1]
  Output : Outport  VectorParamsAs1DForOutWhenUnconnected=off
  wires:
  Input/1 -> Output/1, Signal Specification/1
  Signal Specification/1 -> Matrix Dimension Check/1

== system Model/Adaptive MPC Controller/MPC/MPC Matrix Signal Check U ==
  Input : Inport
  Matrix Dimension Check : S-Function  FunctionName=mpcMatrixSignalCheck  Parameters=blockname, signalname, nrow, ncol, nsteps, isltv  SFunctionDeploymentMode=off  EnableBusSupport=off
  Signal Specification : SignalSpecification  Dimensions=[1 1]
  Output : Outport  VectorParamsAs1DForOutWhenUnconnected=off
  wires:
  Input/1 -> Output/1, Signal Specification/1
  Signal Specification/1 -> Matrix Dimension Check/1

== system Model/Adaptive MPC Controller/MPC/MPC Matrix Signal Check X ==
  Input : Inport
  Matrix Dimension Check : S-Function  FunctionName=mpcMatrixSignalCheck  Parameters=blockname, signalname, nrow, ncol, nsteps, isltv  SFunctionDeploymentMode=off  EnableBusSupport=off
  Signal Specification : SignalSpecification  Dimensions=[4 1]
  Output : Outport  VectorParamsAs1DForOutWhenUnconnected=off
  wires:
  Input/1 -> Output/1, Signal Specification/1
  Signal Specification/1 -> Matrix Dimension Check/1

== system Model/Adaptive MPC Controller/MPC/MPC Matrix Signal Check Y ==
  Input : Inport
  Matrix Dimension Check : S-Function  FunctionName=mpcMatrixSignalCheck  Parameters=blockname, signalname, nrow, ncol, nsteps, isltv  SFunctionDeploymentMode=off  EnableBusSupport=off
  Signal Specification : SignalSpecification  Dimensions=[4 1]
  Output : Outport  VectorParamsAs1DForOutWhenUnconnected=off
  wires:
  Input/1 -> Output/1, Signal Specification/1
  Signal Specification/1 -> Matrix Dimension Check/1

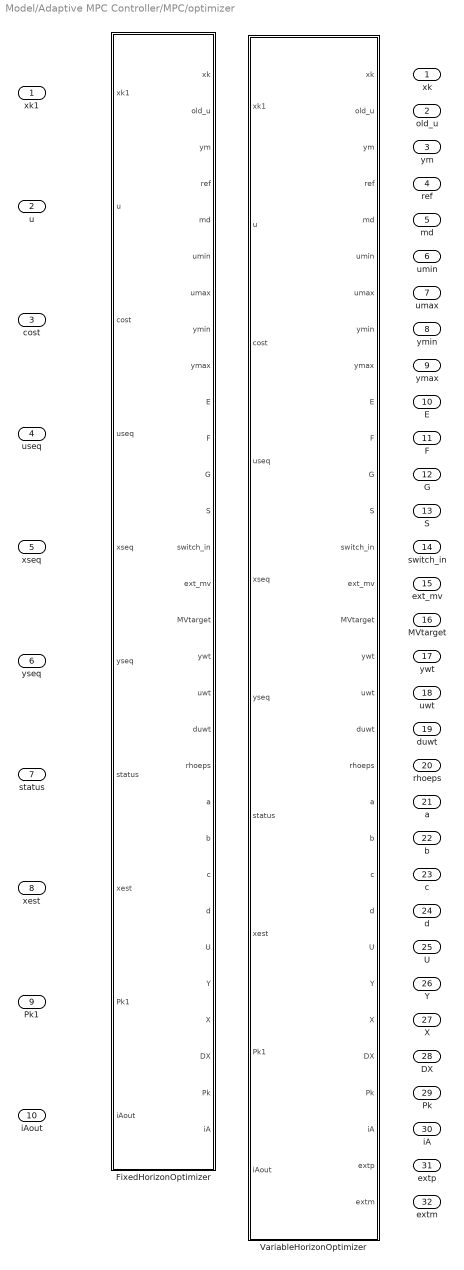
== system Model/Adaptive MPC Controller/MPC/optimizer ==
  "xk " : Inport
  "old_u " : Inport  Port=2
  "ym " : Inport  Port=3
  "ref " : Inport  Port=4
  "md " : Inport  Port=5
  "umin " : Inport  Port=6
  "umax " : Inport  Port=7
  "ymin " : Inport  Port=8
  "ymax " : Inport  Port=9
  "E " : Inport  Port=10
  "F " : Inport  Port=11
  "G " : Inport  Port=12
  "S " : Inport  Port=13
  "switch_in " : Inport  Port=14
  "ext_mv " : Inport  Port=15
  "MVtarget " : Inport  Port=16
  "ywt " : Inport  Port=17
  "uwt " : Inport  Port=18
  "duwt " : Inport  Port=19
  "rhoeps " : Inport  Port=20
  "a " : Inport  Port=21
  "b " : Inport  Port=22
  "c " : Inport  Port=23
  "d " : Inport  Port=24
  "U " : Inport  Port=25
  "Y " : Inport  Port=26
  "X " : Inport  Port=27
  "DX " : Inport  Port=28
  "Pk " : Inport  Port=29
  "iA " : Inport  Port=30
  extp : Inport  Port=31
  extm : Inport  Port=32
  FixedHorizonOptimizer : MATLAB Function  VariantControl=FixedHorizon
  VariableHorizonOptimizer : MATLAB Function  VariantControl=VariableHorizon
  " xk1" : Outport  VectorParamsAs1DForOutWhenUnconnected=off
  " u" : Outport  Port=2  VectorParamsAs1DForOutWhenUnconnected=off
  " cost" : Outport  Port=3  VectorParamsAs1DForOutWhenUnconnected=off
  " useq" : Outport  Port=4  VectorParamsAs1DForOutWhenUnconnected=off
  " xseq" : Outport  Port=5  VectorParamsAs1DForOutWhenUnconnected=off
  " yseq" : Outport  Port=6  VectorParamsAs1DForOutWhenUnconnected=off
  " status" : Outport  Port=7  VectorParamsAs1DForOutWhenUnconnected=off
  " xest" : Outport  Port=8  VectorParamsAs1DForOutWhenUnconnected=off
  " Pk1" : Outport  Port=9  VectorParamsAs1DForOutWhenUnconnected=off
  " iAout" : Outport  Port=10  VectorParamsAs1DForOutWhenUnconnected=off

== system Model/Adaptive MPC Controller1/MPC/MPC Matrix Signal Check A ==
  Input : Inport
  Matrix Dimension Check : S-Function  FunctionName=mpcMatrixSignalCheck  Parameters=blockname, signalname, nrow, ncol, nsteps, isltv  SFunctionDeploymentMode=off  EnableBusSupport=off
  Signal Specification : SignalSpecification  Dimensions=[4 4]
  Output : Outport  VectorParamsAs1DForOutWhenUnconnected=off
  wires:
  Input/1 -> Output/1, Signal Specification/1
  Signal Specification/1 -> Matrix Dimension Check/1

== system Model/Adaptive MPC Controller1/MPC/MPC Matrix Signal Check B ==
  Input : Inport
  Matrix Dimension Check : S-Function  FunctionName=mpcMatrixSignalCheck  Parameters=blockname, signalname, nrow, ncol, nsteps, isltv  SFunctionDeploymentMode=off  EnableBusSupport=off
  Signal Specification : SignalSpecification  Dimensions=[4 1]
  Output : Outport  VectorParamsAs1DForOutWhenUnconnected=off
  wires:
  Input/1 -> Output/1, Signal Specification/1
  Signal Specification/1 -> Matrix Dimension Check/1

== system Model/Adaptive MPC Controller1/MPC/MPC Matrix Signal Check C ==
  Input : Inport
  Matrix Dimension Check : S-Function  FunctionName=mpcMatrixSignalCheck  Parameters=blockname, signalname, nrow, ncol, nsteps, isltv  SFunctionDeploymentMode=off  EnableBusSupport=off
  Signal Specification : SignalSpecification  Dimensions=[4 4]
  Output : Outport  VectorParamsAs1DForOutWhenUnconnected=off
  wires:
  Input/1 -> Output/1, Signal Specification/1
  Signal Specification/1 -> Matrix Dimension Check/1

== system Model/Adaptive MPC Controller1/MPC/MPC Matrix Signal Check D ==
  Input : Inport
  Matrix Dimension Check : S-Function  FunctionName=mpcMatrixSignalCheck  Parameters=blockname, signalname, nrow, ncol, nsteps, isltv  SFunctionDeploymentMode=off  EnableBusSupport=off
  Signal Specification : SignalSpecification  Dimensions=[4 1]
  Output : Outport  VectorParamsAs1DForOutWhenUnconnected=off
  wires:
  Input/1 -> Output/1, Signal Specification/1
  Signal Specification/1 -> Matrix Dimension Check/1

== system Model/Adaptive MPC Controller1/MPC/MPC Matrix Signal Check DX ==
  Input : Inport
  Matrix Dimension Check : S-Function  FunctionName=mpcMatrixSignalCheck  Parameters=blockname, signalname, nrow, ncol, nsteps, isltv  SFunctionDeploymentMode=off  EnableBusSupport=off
  Signal Specification : SignalSpecification  Dimensions=[4 1]
  Output : Outport  VectorParamsAs1DForOutWhenUnconnected=off
  wires:
  Input/1 -> Output/1, Signal Specification/1
  Signal Specification/1 -> Matrix Dimension Check/1

== system Model/Adaptive MPC Controller1/MPC/MPC Matrix Signal Check U ==
  Input : Inport
  Matrix Dimension Check : S-Function  FunctionName=mpcMatrixSignalCheck  Parameters=blockname, signalname, nrow, ncol, nsteps, isltv  SFunctionDeploymentMode=off  EnableBusSupport=off
  Signal Specification : SignalSpecification  Dimensions=[1 1]
  Output : Outport  VectorParamsAs1DForOutWhenUnconnected=off
  wires:
  Input/1 -> Output/1, Signal Specification/1
  Signal Specification/1 -> Matrix Dimension Check/1

== system Model/Adaptive MPC Controller1/MPC/MPC Matrix Signal Check X ==
  Input : Inport
  Matrix Dimension Check : S-Function  FunctionName=mpcMatrixSignalCheck  Parameters=blockname, signalname, nrow, ncol, nsteps, isltv  SFunctionDeploymentMode=off  EnableBusSupport=off
  Signal Specification : SignalSpecification  Dimensions=[4 1]
  Output : Outport  VectorParamsAs1DForOutWhenUnconnected=off
  wires:
  Input/1 -> Output/1, Signal Specification/1
  Signal Specification/1 -> Matrix Dimension Check/1

== system Model/Adaptive MPC Controller1/MPC/MPC Matrix Signal Check Y ==
  Input : Inport
  Matrix Dimension Check : S-Function  FunctionName=mpcMatrixSignalCheck  Parameters=blockname, signalname, nrow, ncol, nsteps, isltv  SFunctionDeploymentMode=off  EnableBusSupport=off
  Signal Specification : SignalSpecification  Dimensions=[4 1]
  Output : Outport  VectorParamsAs1DForOutWhenUnconnected=off
  wires:
  Input/1 -> Output/1, Signal Specification/1
  Signal Specification/1 -> Matrix Dimension Check/1

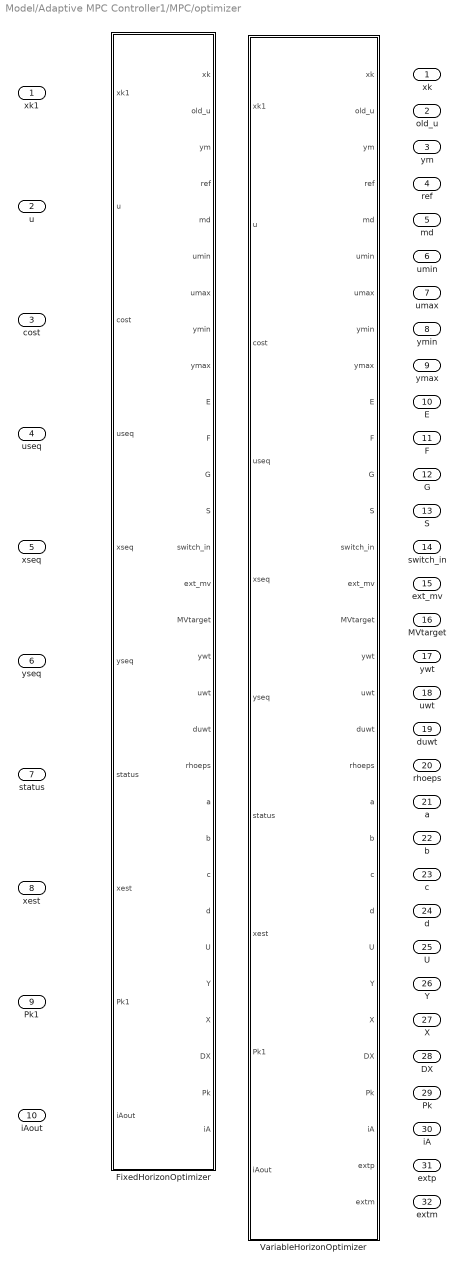
== system Model/Adaptive MPC Controller1/MPC/optimizer ==
  "xk " : Inport
  "old_u " : Inport  Port=2
  "ym " : Inport  Port=3
  "ref " : Inport  Port=4
  "md " : Inport  Port=5
  "umin " : Inport  Port=6
  "umax " : Inport  Port=7
  "ymin " : Inport  Port=8
  "ymax " : Inport  Port=9
  "E " : Inport  Port=10
  "F " : Inport  Port=11
  "G " : Inport  Port=12
  "S " : Inport  Port=13
  "switch_in " : Inport  Port=14
  "ext_mv " : Inport  Port=15
  "MVtarget " : Inport  Port=16
  "ywt " : Inport  Port=17
  "uwt " : Inport  Port=18
  "duwt " : Inport  Port=19
  "rhoeps " : Inport  Port=20
  "a " : Inport  Port=21
  "b " : Inport  Port=22
  "c " : Inport  Port=23
  "d " : Inport  Port=24
  "U " : Inport  Port=25
  "Y " : Inport  Port=26
  "X " : Inport  Port=27
  "DX " : Inport  Port=28
  "Pk " : Inport  Port=29
  "iA " : Inport  Port=30
  extp : Inport  Port=31
  extm : Inport  Port=32
  FixedHorizonOptimizer : MATLAB Function  VariantControl=FixedHorizon
  VariableHorizonOptimizer : MATLAB Function  VariantControl=VariableHorizon
  " xk1" : Outport  VectorParamsAs1DForOutWhenUnconnected=off
  " u" : Outport  Port=2  VectorParamsAs1DForOutWhenUnconnected=off
  " cost" : Outport  Port=3  VectorParamsAs1DForOutWhenUnconnected=off
  " useq" : Outport  Port=4  VectorParamsAs1DForOutWhenUnconnected=off
  " xseq" : Outport  Port=5  VectorParamsAs1DForOutWhenUnconnected=off
  " yseq" : Outport  Port=6  VectorParamsAs1DForOutWhenUnconnected=off
  " status" : Outport  Port=7  VectorParamsAs1DForOutWhenUnconnected=off
  " xest" : Outport  Port=8  VectorParamsAs1DForOutWhenUnconnected=off
  " Pk1" : Outport  Port=9  VectorParamsAs1DForOutWhenUnconnected=off
  " iAout" : Outport  Port=10  VectorParamsAs1DForOutWhenUnconnected=off

== system Model/Adaptive MPC Controller2/MPC/MPC Matrix Signal Check A ==
  Input : Inport
  Matrix Dimension Check : S-Function  FunctionName=mpcMatrixSignalCheck  Parameters=blockname, signalname, nrow, ncol, nsteps, isltv  SFunctionDeploymentMode=off  EnableBusSupport=off
  Signal Specification : SignalSpecification  Dimensions=[4 4]
  Output : Outport  VectorParamsAs1DForOutWhenUnconnected=off
  wires:
  Input/1 -> Output/1, Signal Specification/1
  Signal Specification/1 -> Matrix Dimension Check/1

== system Model/Adaptive MPC Controller2/MPC/MPC Matrix Signal Check B ==
  Input : Inport
  Matrix Dimension Check : S-Function  FunctionName=mpcMatrixSignalCheck  Parameters=blockname, signalname, nrow, ncol, nsteps, isltv  SFunctionDeploymentMode=off  EnableBusSupport=off
  Signal Specification : SignalSpecification  Dimensions=[4 1]
  Output : Outport  VectorParamsAs1DForOutWhenUnconnected=off
  wires:
  Input/1 -> Output/1, Signal Specification/1
  Signal Specification/1 -> Matrix Dimension Check/1

== system Model/Adaptive MPC Controller2/MPC/MPC Matrix Signal Check C ==
  Input : Inport
  Matrix Dimension Check : S-Function  FunctionName=mpcMatrixSignalCheck  Parameters=blockname, signalname, nrow, ncol, nsteps, isltv  SFunctionDeploymentMode=off  EnableBusSupport=off
  Signal Specification : SignalSpecification  Dimensions=[4 4]
  Output : Outport  VectorParamsAs1DForOutWhenUnconnected=off
  wires:
  Input/1 -> Output/1, Signal Specification/1
  Signal Specification/1 -> Matrix Dimension Check/1

== system Model/Adaptive MPC Controller2/MPC/MPC Matrix Signal Check D ==
  Input : Inport
  Matrix Dimension Check : S-Function  FunctionName=mpcMatrixSignalCheck  Parameters=blockname, signalname, nrow, ncol, nsteps, isltv  SFunctionDeploymentMode=off  EnableBusSupport=off
  Signal Specification : SignalSpecification  Dimensions=[4 1]
  Output : Outport  VectorParamsAs1DForOutWhenUnconnected=off
  wires:
  Input/1 -> Output/1, Signal Specification/1
  Signal Specification/1 -> Matrix Dimension Check/1

== system Model/Adaptive MPC Controller2/MPC/MPC Matrix Signal Check DX ==
  Input : Inport
  Matrix Dimension Check : S-Function  FunctionName=mpcMatrixSignalCheck  Parameters=blockname, signalname, nrow, ncol, nsteps, isltv  SFunctionDeploymentMode=off  EnableBusSupport=off
  Signal Specification : SignalSpecification  Dimensions=[4 1]
  Output : Outport  VectorParamsAs1DForOutWhenUnconnected=off
  wires:
  Input/1 -> Output/1, Signal Specification/1
  Signal Specification/1 -> Matrix Dimension Check/1
